simulink model "rlc"  (R2016a)
settings: Solver=VariableStepAuto  StartTime=0.0  StopTime=3  RelTol=1e-3
values from neighbouring files (symbols this model uses):
  Llsr = sigma*Ls    [normalOp.m]    (also in stationary_from_eq.m)
  Lmr = (1-sigma)*Ls    [normalOp.m]    (also in stationary_from_eq.m)
  Rrr = Rr *a*a    [normalOp.m]    (also in stationary_from_eq.m)
  Rs = 1.725    [motor4_workspace.mat]    (also in motor_wrapper.m = obj.Rs; scim_verifier.m = obj.motor.getRs(); setMotorParams.m; stationary_class.m = obj.Rs)
libraries: powerlib x11
settings Model: Creator=ebenera  LastModifiedBy=ebenera

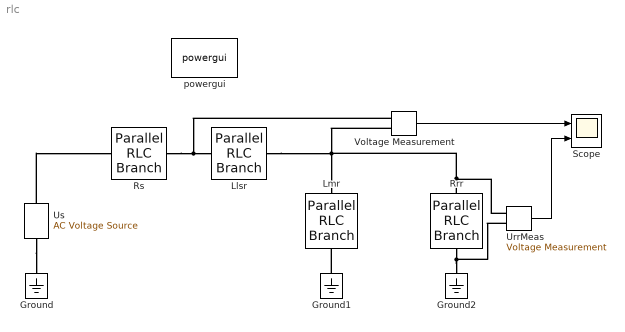
== system rlc ==
  Ground : powerlib/Elements/Ground  LConnTagsString=a
  Ground1 : powerlib/Elements/Ground  LConnTagsString=a
  Ground2 : powerlib/Elements/Ground  LConnTagsString=a
  Llsr : powerlib/Elements/Parallel RLC Branch  LConnTagsString=a  RConnTagsString=__new0  BranchType=L  Resistance=2  Inductance=Llsr  SetiL0=off  InitialCurrent=0  Capacitance=1e-6  Setx0=off  InitialVoltage=0  Measurements=None
  Lmr : powerlib/Elements/Parallel RLC Branch  LConnTagsString=a  RConnTagsString=__new0  BranchType=L  Resistance=2  Inductance=Lmr  SetiL0=off  InitialCurrent=0  Capacitance=1e-6  Setx0=off  InitialVoltage=0  Measurements=None
  Rrr : powerlib/Elements/Parallel RLC Branch  LConnTagsString=a  RConnTagsString=__new0  BranchType=R  Resistance=Rrr  Inductance=0  SetiL0=off  InitialCurrent=0  Capacitance=0  Setx0=off  InitialVoltage=0  Measurements=None
  Rs : powerlib/Elements/Parallel RLC Branch  LConnTagsString=a  RConnTagsString=__new0  BranchType=R  Resistance=Rs  Inductance=0  SetiL0=off  InitialCurrent=0  Capacitance=0  Setx0=off  InitialVoltage=0  Measurements=None
  Scope : Scope  NumInputPorts=2
  UrrMeas : powerlib/Measurements/Voltage Measurement  PhasorSimulation=off  OutputType=Complex  PSBequivalent=0
  Us : powerlib/Electrical Sources/AC Voltage Source  Amplitude=100  Phase=0  Frequency=om1/2/pi  SampleTime=0  Measurements=None  BusType=swing  Pref=10e3  Qref=0  Qmin=-inf  Qmax=+inf
  Voltage Measurement : powerlib/Measurements/Voltage Measurement  PhasorSimulation=off  OutputType=Complex  PSBequivalent=0
  powergui : powerlib/powergui  Priority=1  SimulationMode=Continuous  SolverType=Tustin/Backward Euler (TBE)  SampleTime=50e-6  frequency=60  SPID=off  DisableSnubberDevices=off  DisableRonSwitches=off  DisableVfSwitches=off  SwTol=0  DisplayEquations=off  Interpol=off  ExternalGateDelay=off  methode=off  Ts=10  FunctionMessages=off  echomessages=off  HookPort=off  EnableUseOfTLC=off  x0status=blocks  frequencyindice=23.8732414637843  Pbase=100e6  ErrMax=1e-4  Iterations=50  UnitsV=kV  UnitsW=MW  buscounter=0  RestoreLinks=warning  ResistiveCurrentMeasurement=off  Frange=[0:2:500]  Ylog=off  Xlog=on  ShowGrid=off  save=off  variable=ZData  structure=0  ZoomFFT=off  StartTime=0.0  cycles=1  DisplayStyle=1  fundamental=60  FreqAxis=off  MaxFrequency=1000  frequencyindicesteady=1  RmsSteady=1  display=off
  wires:
  Voltage Measurement/1 -> Scope/1
  UrrMeas/1 -> Scope/2
  connections:
  Rs/RConn1 -- Voltage Measurement/LConn1 -- Llsr/LConn1
  Us/RConn1 -- Rs/LConn1
  Us/LConn1 -- Ground/LConn1
  Llsr/RConn1 -- UrrMeas/LConn1 -- Rrr/LConn1 -- Lmr/LConn1 -- Voltage Measurement/LConn2
  Ground1/LConn1 -- Lmr/RConn1
  Rrr/RConn1 -- UrrMeas/LConn2 -- Ground2/LConn1
